simulink model "WEankle_controllerMaarten_2018"  (R2018b)
settings: Solver=FixedStepDiscrete  StartTime=0.0  StopTime=inf  FixedStep=sampleTime  RelTol=1e-3
PreLoadFcn:
  | init
undefined symbols (not defined in the file or in its folder): DiscIntNeverNeededParam, forceplate, Joint_params, sampleTime
libraries: simulink x21, WE2_library x9, dspsigops x6, dspfdesign x3
(part 4 of 4)

== matlab function WEankle_controllerMaarten_2018/FromActuators/RA/ToJointTorque/MATLAB Function ==
  data: u input; y output int32; counts_rev input; dowrap input
function y = wrapAroundZero(u, counts_rev, dowrap)
%#codegen
%
% Depending on the value of dowrap, this function does the following:
% dowrap == 0 -> pass u unchanged; i.e., y=u; (normal case)
%                This implies that at u=0 a 'jump' of one full turn is
%                seen. If 0 is not within the range of motion, this is
%                acceptable (you always have a jump somewhere).
% dowrap == 1 -> Interpret u as a couts_rev-size _signed_ integer, and output 
%                the value of this signed integer as y. In this case, the
%                'jump' is at counts_rev/2. Use this case when 0 is within
%                the range of motion (and counts_rev/2 is outside it).
% Since the range of motion of each joint is less than pi, there is always
% one of the above possibilities that can be chosen (in other words, there
% is always at least one of [0, counts_rev/2] outside the range of motion).
%                
if ~dowrap
    y = int32(u); % The counts_rev is in our case 2^20, so this gives no danger of being outside the range of an int32.
                  % (note that u is a uint32)
else
    % Do the wrapping
    if u <= abs(counts_rev)/2
        y=int32(u);
    else
        y=int32(u) - int32(abs(counts_rev));
    end;
end;

== matlab function WEankle_controllerMaarten_2018/FromActuators/RA/ToJointTorque/MATLAB Function1 ==
  data: u input; y output int32; counts_rev input; dowrap input
function y = wrapAroundZero(u, counts_rev, dowrap)
%#codegen
%
% Depending on the value of dowrap, this function does the following:
% dowrap == 0 -> pass u unchanged; i.e., y=u; (normal case)
%                This implies that at u=0 a 'jump' of one full turn is
%                seen. If 0 is not within the range of motion, this is
%                acceptable (you always have a jump somewhere).
% dowrap == 1 -> Interpret u as a couts_rev-size _signed_ integer, and output 
%                the value of this signed integer as y. In this case, the
%                'jump' is at counts_rev/2. Use this case when 0 is within
%                the range of motion (and counts_rev/2 is outside it).
% Since the range of motion of each joint is less than pi, there is always
% one of the above possibilities that can be chosen (in other words, there
% is always at least one of [0, counts_rev/2] outside the range of motion).
%                
if ~dowrap
    y = int32(u); % The counts_rev is in our case 2^20, so this gives no danger of being outside the range of an int32.
                  % (note that u is a uint32)
else
    % Do the wrapping
    if u <= abs(counts_rev)/2
        y=int32(u);
    else
        y=int32(u) - int32(abs(counts_rev));
    end;
end;

== matlab function WEankle_controllerMaarten_2018/FromActuators/RA/ToMotorAngle_rad/MotorAngle ==
  data: pos input; gearboxRatio parameter; encoderCounts_rev parameter; pos_mot_rad output; JointAngle_rad input; SpringDeflection_rad input; Calibrate input
function pos_mot_rad  = ...
    PosActValDecode(pos, gearboxRatio, encoderCounts_rev, JointAngle_rad, SpringDeflection_rad, Calibrate)
%#codegen
%
% The output is the motor angle, converted to AFTER the gearbox
% (thus the value you get here is equal to the true rotor angle divided by
% the gearbox ratio). It has the same order of magnitude, and is directly
% comparable to the joint angle and spring angle.

% This block includes calibration such that (ideally) the motor angle is
% zero when the joint angle and spring deflection are zero as well. Before
% the calibration has occurred, the output of this function is -10*. This
% is chosen such that the value is always outside the allowed motor angle
% range; this prevents the drive from being allowed to turn on (since we
% have no multiple-rotation parts, we can never have a value larger than
% -2pi. Chose -10 because it is not ridiculously large so the vertical
% scaling of graphs will not be affected that severely.
% 
%
% * I wanted to use -inf as starting function, but I'm not sure whether
%   that will be handled correctly in all cases.

persistent isCalibrated;
persistent offset;

if isempty(isCalibrated)
    isCalibrated = 0;
    offset = 0;
end

pos_inc = double(pos);

if Calibrate
    pos_mot_rad_temp = pos_inc * 2*pi / (encoderCounts_rev * gearboxRatio); % The angle we read from the motor encoder
    target_pos_mot_rad = JointAngle_rad + SpringDeflection_rad; % This is what we should read
    offset = target_pos_mot_rad - pos_mot_rad_temp;
    isCalibrated = 1;
end

if isCalibrated
    pos_mot_rad = pos_inc * 2*pi / (encoderCounts_rev * gearboxRatio) + offset;
else
    pos_mot_rad = -10;
end

== matlab function WEankle_controllerMaarten_2018/Ankle Controller/COMverror and perturbation/COMvError/Signal learner/MATLAB Function1 ==
  data: t input; trigger input; signal input; signal_learned output; n_strides_ output; n_ output; m_ output; output_duration_ output; n_rep input; perturbation output; threshPert input; DataLost input; ShutDown output
function [signal_learned,n_strides_,n_,m_,output_duration_,perturbation,ShutDown] = signal_learner(t,trigger,signal,n_rep,threshPert,DataLost)
%     n_rep = how many signals period will be averaged
    n_storage = 2000; %stored signal will be 2000 elements long. playback will be interpolated
    n_buffer_size = 4000; %can maximally read 4000;
    perturbation = 0;
    ShutDown = 0; %No trigger the controller if DataLost or if we are in the first n_rep strides
    persistent n %elements of vector
    persistent n_strides % total number of strides
    persistent m %Pointer for recording each stride in buffer (1:n_rep)
    persistent t0 % moment in time of last stride
    persistent last_buffer
    persistent output_signal_buffer
    persistent output_signal
    persistent output_duration
    persistent output_duration_buffer
    persistent maximums
    persistent MaxAver
%     persistent Perturbation
    if isempty(n)
       n = 1;
       m = 1;
       t0 = 0;
       last_buffer = zeros(1,n_buffer_size);
       output_signal_buffer = zeros(n_rep,n_storage);
       output_signal = zeros(1,n_storage);
       output_duration_buffer = zeros(n_rep,1);
       n_strides = 0;
       output_duration = 1;%1.0;
       % Added Cristina
%        Perturbation = 0;
       maximums = 200*ones(n_rep,1); %to store the maximums of previous steps
       MaxAver = 200; % This number multiply by 1.5 is the one above which a perturbation is supposed to happen,
%     and thereby, that step will be excluded to calculate the mean
    end
if ~DataLost
    t_rel = t-t0;
    if (trigger && t_rel > 0.1) %if trigger happens, note down the absolute time when that was
        n_strides = n_strides+1; %counting number of strides
        last_stride_duration = t-t0;

        t0 = t; %Reset the moment when the last stride happened
        %% Added Cristina
        % See if there was a perturbation in the last step
        Perturbation = 0; % Init perturbation in the last step
        leng = length(last_buffer(1:min([n,n_buffer_size])));
        for i = 1:leng
            element = last_buffer(i);
            if element > 1.5*MaxAver % A perturbation was detected in the last step
                Perturbation = 1;
            end
        end
        
        %% Changed Cristina
        if n_strides >= 3 
            if (last_stride_duration > 0.5*output_duration)% to avoid false triggers
                enter = 1;
            else
                enter = 0;
            end
        else
            enter = 1;
        end
        if (last_stride_duration > 0) && enter % otherwise failure at start or false trigger  % > 0) %otherwise failure at start
            % If there was no perturbation, take that step into account.
            % Otherwise, exclude it
            if ~Perturbation %in the last step
                %interpolate regardless of last duration to n_storage elements
                output_signal_buffer(m,:) = ...
                    interp1(...
                    linspace(0,last_stride_duration,n),... %vector of n elements
                    last_buffer(1:min([n,n_buffer_size])),... %only read up to incl. n elements, if bigger than n_buffer size, then we need to limit.
                    linspace(0,last_stride_duration,n_storage)); %remap that to a new 'x' with n_storage elements
                output_signal = mean(output_signal_buffer); %averages over n_rep stored signals
                
                output_duration_buffer(m) = last_stride_duration;
                output_duration = mean(output_duration_buffer); %duration is average of last n_rep times
                
                maximums(m) = max(last_buffer(1:min([n,n_buffer_size]))); %store the new maximum of current step
                MaxAver = mean(maximums); %calculate the average of maximums found in the last n_rep
                
                m = m+1;
                if m > n_rep 
                    m = 1;
                end
            end
            if (n_strides <= n_rep)
                output_duration = last_stride_duration;
            end
            %last_buffer = zeros() %is not required due to 1:n
            n = 1;
        end
    end
end  
if ~DataLost
    %% process input
    t_rel = t-t0;
    last_buffer(min([n n_buffer_size])) = signal;

    %% generate output
    fractional_index = t_rel/output_duration * (n_storage-1);
    rounded_index = min([1+floor(fractional_index),n_storage]); %cannot overflow
    fraction = 1+fractional_index - rounded_index;
    
    %linearly interpolate
    if (rounded_index >= n_storage - 1)
        signal_learned = output_signal(n_storage-1);
    else
        signal_learned = output_signal(rounded_index)*(1-fraction) + output_signal(rounded_index+1)*fraction;
    end

    %debug output
    n_strides_ = n_strides;
    n_ = n;
    m_ = m;
    output_duration_ = output_duration;
    if signal > threshPert*MaxAver
        perturbation = 1;
    end
else
    %debug output
    n_strides_ = n_strides;
    n_ = n;
    m_ = m;
    output_duration_ = output_duration;
    perturbation = 0;
    signal_learned = 0;
end

%do not output anything learned in first n_rep strides.
if (n_strides <= n_rep) || DataLost
    signal_learned = 0;
    output_duration_ = 0;%last_stride_duration;
    ShutDown = 1;
end
if ~DataLost
    %shift signal storage pointer, avoid overflow
    n = n+1;
else
    n = 1;
end
end

== matlab function WEankle_controllerMaarten_2018/Ankle Controller/AnkleControllerGeyer1/Muscle Geometry ==
  data: q input; lMT output; dM output; qOffsetLeft input; qOffsetRight input
function [lMT,dM] = GetMuscleGeometry_Simulink(q,qOffsetLeft,qOffsetRight)
% GetMuscleGeometry is a function that uses polynomials to evaluate the muscle-tendon
% lengths, velocities and  moment arms as a function of the joint angles and velocities.
% Inputs:
%   - q: vector with joint angles
% Outputs:
%   - lMT: muscle-tendon length
%   - dM: moment arm

lMT = zeros(4,1);
dM = zeros(4,1);

qrel = q - [qOffsetLeft; qOffsetRight];

for i = 1:length(qrel)
    if  qrel(i) < -15*pi/180
        qrel(i) = -15*pi/180;
    end
    if  qrel(i) > 15*pi/180
        qrel(i) = 15*pi/180;
    end
end

% use matlab function to get muscle geometry
[lMT_Left,dM_Left] = GetMuscleGeometry_LengthOnly(-qrel(1));
[lMT_Right,dM_Right] = GetMuscleGeometry_LengthOnly(-qrel(2));

lMT = [lMT_Left; lMT_Right];
dM = [dM_Left; dM_Right];

end

== matlab function WEankle_controllerMaarten_2018/GetAnkleAngleStanding/MATLAB Function ==
  data: q input; qOff output; start input; caltime_s input
function qOff = EncoderOffset_GeyerModel(q, start, caltime_s)
% q = joint angle
% start = boolean indicate start callibration is triggered
% caltime_s = total callibration time

qOff = f_EncoderOffset_GeyerModel(q,start,caltime_s);

== matlab function WEankle_controllerMaarten_2018/GetAnkleAngleStanding/MATLAB Function1 ==
  data: q input; qOff output; start input; caltime_s input
function qOff = EncoderOffset_GeyerModel(q, start, caltime_s)
% q = joint angle
% start = boolean indicate start callibration is triggered
% caltime_s = total callibration time

qOff = f_EncoderOffset_GeyerModel(q,start,caltime_s);

== matlab function WEankle_controllerMaarten_2018/Ankle Controller/MATLAB Function9 ==
  data: tau_Reflex input; tau_ReflexUnp input; tau_Left output; BodyMass input; BodyLength input; tau_Right output; MaxTorque input; TorqueScale input; ControlType input
function [tau_Left, tau_Right]  = DesiredExoMoment(tau_Reflex, tau_ReflexUnp,...
    BodyMass, BodyLength, MaxTorque, TorqueScale,ControlType)
%DesiredExoMoment switched between control types and selects the desired
%exo moment for the left and right leg

[tau_Left, tau_Right]  = f_DesiredExoMoment(tau_Reflex, tau_ReflexUnp,...
    BodyMass, BodyLength, MaxTorque, TorqueScale,ControlType);

== matlab function WEankle_controllerMaarten_2018/Ankle Controller/AnkleControllerGeyer/Muscle Geometry ==
  data: q input; lMT output; dM output; qOffsetLeft input; qOffsetRight input
function [lMT,dM] = GetMuscleGeometry_Simulink(q,qOffsetLeft,qOffsetRight)
% GetMuscleGeometry is a function that uses polynomials to evaluate the muscle-tendon
% lengths, velocities and  moment arms as a function of the joint angles and velocities.
% Inputs:
%   - q: vector with joint angles
% Outputs:
%   - lMT: muscle-tendon length
%   - dM: moment arm

lMT = zeros(4,1);
dM = zeros(4,1);

qrel = q - [qOffsetLeft; qOffsetRight];

for i = 1:length(qrel)
    if  qrel(i) < -15*pi/180
        qrel(i) = -15*pi/180;
    end
    if  qrel(i) > 15*pi/180
        qrel(i) = 15*pi/180;
    end
end

% use matlab function to get muscle geometry
[lMT_Left,dM_Left] = GetMuscleGeometry_LengthOnly(-qrel(1));
[lMT_Right,dM_Right] = GetMuscleGeometry_LengthOnly(-qrel(2));

lMT = [lMT_Left; lMT_Right];
dM = [dM_Left; dM_Right];

end

== matlab function WEankle_controllerMaarten_2018/Ankle Controller/AnkleControllerGeyer/MATLAB Function1 ==
  data: GRFy_Left input; GRFy_Right input; e output; Ftilde input; lMtilde input; COMd input; SoleusGains input; TibialisGains input; BodyMass input
function e  = GeyerAnkleModel_Simulink(GRFy_Left,GRFy_Right,Ftilde,lMtilde, COMd, SoleusGains, TibialisGains, BodyMass )
% input arguments:

% extract structure with gains from gains vector (makes it easier to read)
Gains = ExtractGains(SoleusGains,TibialisGains);

% compute excitations based on feedback models
[eLeft] = GeyerAnkle(GRFy_Left,Gains,Ftilde(1),lMtilde(2),COMd, BodyMass);
[eRight] = GeyerAnkle(GRFy_Right,Gains,Ftilde(3),lMtilde(4),COMd, BodyMass);

% vector with excitations
e =[eLeft; eRight];

== matlab function WEankle_controllerMaarten_2018/Ankle Controller/AnkleControllerGeyer/ActivationDynamics1 ==
  data: e input; dadt output; a input
function dadt = ActDyn(e,a)

% See publication (DeGroote2016), equations 1-2, for more details
% (note tanh implementation mainly needed for gradient based optimization.
% Not needed in the actual controller. (I decided to keep it so that the
% dynamics of the parameter estimation and the controller are exactly the
% same

% tact = 0.02;
% tdeact = 0.04;

% contraction dynamics with smooth transition
% b = 0.001;
% d1 = 1./(tact.*(0.5+1.5*a));
% d2 = (0.5+1.5*a)./tdeact;
% f = 0.5*tanh(b*(e-a));
% dadt = (d1.*(f+0.5) + d2.*(-f+0.5)).*(e-a);

% try explicit version of contraction dynamics ( error in twincat with
% smooth version
% dadt = zeros(4,1);
% for i=1:length(a)
%     if a(i) < e(i)
%         tau_sel = tact;
%     else
%         tau_sel = tdeact;
%     end
%     dadt(i) = (e(i)-a(i))./ tau_sel;    
% end

% dadt = zeros(4,1);
% for i=1:length(a)   
%     dadt(i) = (e(i)-a(i))./ 0.03;    
% end

dadt = (e-a)./0.03;

== matlab function WEankle_controllerMaarten_2018/Ankle Controller/AnkleControllerGeyer/ContractionDynamics1 ==
  data: a input; dlMdt output; lMtilde input; lMT input; F output; Fce_tilde output
function [dlMdt, F , Fce_tilde] = ContractionDynamics_Simulink(a,lMtilde,lMT)
% ContractionDynamics_Simulink Simulates contraction dynamics

% Muscle contraction dynamics left leg
[dlMdt_Left, F_Left , Fce_tilde_Left] = MuscleContractionDynamics(a(1:2),lMtilde(1:2),lMT(1:2));
 
% Muscle contraction dynamics right leg
[dlMdt_Right, F_Right , Fce_tilde_Right] = MuscleContractionDynamics(a(3:4),lMtilde(3:4),lMT(3:4));

% combine vectors
dlMdt = [dlMdt_Left; dlMdt_Right];
F = [F_Left; F_Right];
Fce_tilde = [Fce_tilde_Left; Fce_tilde_Right];

== matlab function WEankle_controllerMaarten_2018/Ankle Controller/AnkleControllerGeyer/ContractionDynamics2 ==
  data: F input; tauModel output; dM input
function tauModel  = ComputeJointMoment(F,dM)

% matlab function to compute muscle contraction dynamics
tauLeft = dM(1).*F(1) + dM(2).*F(2);
tauRight = dM(3).*F(3) + dM(4).*F(4);
tauModel = [tauLeft; tauRight];

== matlab function WEankle_controllerMaarten_2018/Ankle Controller/MATLAB Function3 ==
  data: e0 input; G input; SolGains output; COMd input
function SolGains  = CombineSoleusGains(e0,G,COMd)
% input arguments:

SolGains = [e0; G; COMd];

== matlab function WEankle_controllerMaarten_2018/Ankle Controller/MATLAB Function4 ==
  data: e0 input; G input; loff input; GSol input; TibGains output; COMd input
function TibGains  = CombineTibGains(e0,G,loff,GSol,COMd)
% input arguments:

TibGains = [e0; G; loff; GSol; COMd];
